simulink model "threeDOFmodel"  (R2018b)
settings: Solver=VariableStepAuto  StartTime=0.0  StopTime=inf  RelTol=1e-3
libraries: robotlib x15, autolibshared x2
settings Model: Creator=ckreienk  LastModifiedBy=ckreienk

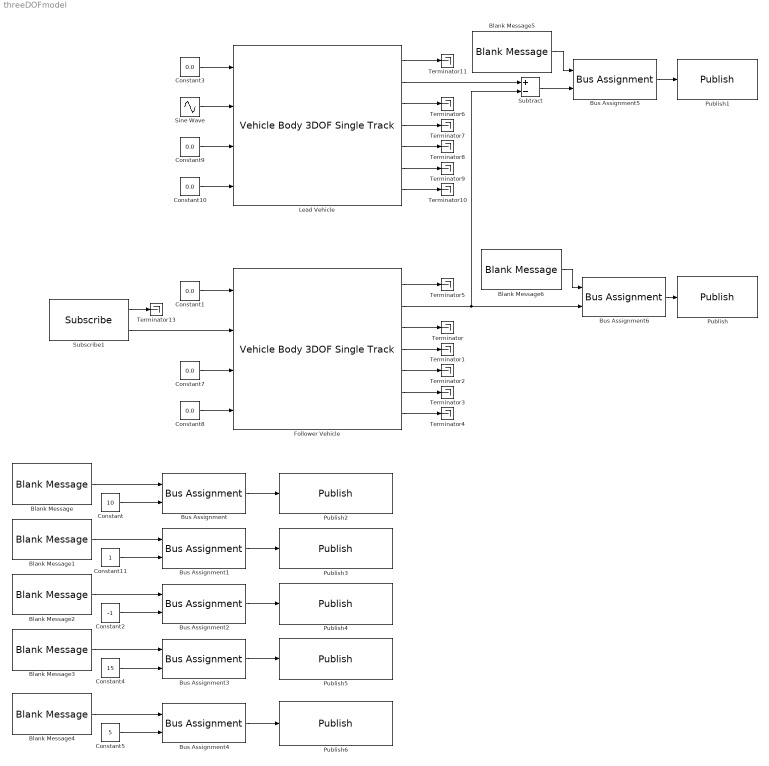
== system threeDOFmodel ==
  Blank Message{,1..6} (7 alike) : robotlib/Blank Message  messageClass=Message  entityType=geometry_msgs/Point  messageType=geometry_msgs/Point  SampleTime=inf
      settings: SourceProductBaseCode=RO
  Bus Assignment{,1..6} (7 alike) : BusAssignment  AssignedSignals=X
  Constant : Constant  Value=10
  Constant{1,3,7..10} (6 alike) : Constant  Value=0.0
  Constant11 : Constant
  Constant2 : Constant  Value=-1
  Constant4 : Constant  Value=15
  Constant5 : Constant  Value=5
  Follower Vehicle : autolibshared/Vehicle Body 3DOF Single Track  trackMode=Dual  inputMode=External longitudinal velocity  frontSteerMode=on  rearSteerMode=off  windMode=off  muMode=on  extFMode=on  extMMode=off  aMode=2  NF=2  NR=2  m=2000  a=1.4  b=1.6  h=0.35  X_o=0  xdot_o=0  CalphaMode=off  sigmaMode=on  d=0  w=[1.4,1.4]  Cy_f=12e3  Cy_r=11e3  sigma_f=.1  sigma_r=.1  alpha_f_brk=[-.1 .1]  Cy_f_data=[-9e3 9e3]  alpha_r_brk=[-.1 .1]  Cy_r_data=[-9e3 9e3]  Y_o=0  ydot_o=0  Izz=4000  psi_o=0  r_o=0  Af=2  Cd=.3  Cl=.1  Cpm=.1  beta_w=[0:0.01:0.3]  Cs=[0:0.03:0.9]  Cym=[0:0.01:0.3]  Pabs=101325  Tair=273  g=9.81  mu=1  xdot_tol=.01  Fznom=5000  Fxtire_sat=7e4  Fytire_sat=7e4  longOff=0  latOff=0  vertOff=0
      settings: SourceProductName=Powertrain Blockset  SourceProductBaseCode=PW
  Lead Vehicle : autolibshared/Vehicle Body 3DOF Single Track  trackMode=Dual  inputMode=External longitudinal velocity  frontSteerMode=on  rearSteerMode=off  windMode=off  muMode=on  extFMode=on  extMMode=off  aMode=2  NF=2  NR=2  m=2000  a=1.4  b=1.6  h=0.35  X_o=0  xdot_o=0  CalphaMode=off  sigmaMode=on  d=0  w=[1.4,1.4]  Cy_f=12e3  Cy_r=11e3  sigma_f=.1  sigma_r=.1  alpha_f_brk=[-.1 .1]  Cy_f_data=[-9e3 9e3]  alpha_r_brk=[-.1 .1]  Cy_r_data=[-9e3 9e3]  Y_o=0  ydot_o=0  Izz=4000  psi_o=0  r_o=0  Af=2  Cd=.3  Cl=.1  Cpm=.1  beta_w=[0:0.01:0.3]  Cs=[0:0.03:0.9]  Cym=[0:0.01:0.3]  Pabs=101325  Tair=273  g=9.81  mu=1  xdot_tol=.01  Fznom=5000  Fxtire_sat=7e4  Fytire_sat=7e4  longOff=0  latOff=0  vertOff=0
      settings: SourceProductName=Powertrain Blockset  SourceProductBaseCode=PW
  Publish : robotlib/Publish  topicSource=Specify your own  topic=vel  messageType=geometry_msgs/Point  messageQueueLength=1
      settings: SourceProductBaseCode=RO
  Publish1 : robotlib/Publish  topicSource=Specify your own  topic=kalmanFilter/vel  messageType=geometry_msgs/Point  messageQueueLength=1
      settings: SourceProductBaseCode=RO
  Publish2 : robotlib/Publish  topicSource=Specify your own  topic=/smoothupparams/max_speed  messageType=geometry_msgs/Point  messageQueueLength=1
      settings: SourceProductBaseCode=RO
  Publish3 : robotlib/Publish  topicSource=Specify your own  topic=/smoothupparams/max_accel  messageType=geometry_msgs/Point  messageQueueLength=1
      settings: SourceProductBaseCode=RO
  Publish4 : robotlib/Publish  topicSource=Specify your own  topic=/smoothupparams/max_decel  messageType=geometry_msgs/Point  messageQueueLength=1
      settings: SourceProductBaseCode=RO
  Publish5 : robotlib/Publish  topicSource=Specify your own  topic=reference_vel  messageType=geometry_msgs/Point  messageQueueLength=1
      settings: SourceProductBaseCode=RO
  Publish6 : robotlib/Publish  topicSource=Specify your own  topic=kalmanFilter/dist  messageType=geometry_msgs/Point  messageQueueLength=1
      settings: SourceProductBaseCode=RO
  Sine Wave : Sin  Amplitude=3  Bias=3  Frequency=3  SampleTime=0
  Subscribe1 : robotlib/Subscribe  topicSource=Specify your own  topic=cmd_vel_wrench  messageType=geometry_msgs/Point  sampleTime=-1  messageQueueLength=1
      settings: SourceProductBaseCode=RO
  Subtract : Sum  Inputs=+-
  Terminator{,1..11,13} (13 alike) : Terminator
  wires:
  Subscribe1/2 -> Follower Vehicle/2
  Constant1/1 -> Follower Vehicle/1
  Follower Vehicle/7 -> Terminator4/1
  Follower Vehicle/6 -> Terminator3/1
  Follower Vehicle/5 -> Terminator2/1
  Follower Vehicle/4 -> Terminator1/1
  Follower Vehicle/3 -> Terminator/1
  Follower Vehicle/1 -> Terminator5/1
  Lead Vehicle/1 -> Terminator11/1
  Lead Vehicle/3 -> Terminator6/1
  Lead Vehicle/4 -> Terminator7/1
  Lead Vehicle/5 -> Terminator8/1
  Lead Vehicle/6 -> Terminator9/1
  Lead Vehicle/7 -> Terminator10/1
  Constant3/1 -> Lead Vehicle/1
  Subscribe1/1 -> Terminator13/1
  Sine Wave/1 -> Lead Vehicle/2
  Bus Assignment5/1 -> Publish1/1
  Constant7/1 -> Follower Vehicle/3
  Constant8/1 -> Follower Vehicle/4
  Constant9/1 -> Lead Vehicle/3
  Constant10/1 -> Lead Vehicle/4
  Bus Assignment/1 -> Publish2/1
  Blank Message/1 -> Bus Assignment/1
  Constant/1 -> Bus Assignment/2
  Constant11/1 -> Bus Assignment1/2
  Blank Message1/1 -> Bus Assignment1/1
  Constant2/1 -> Bus Assignment2/2
  Constant4/1 -> Bus Assignment3/2
  Constant5/1 -> Bus Assignment4/2
  Bus Assignment4/1 -> Publish6/1
  Blank Message4/1 -> Bus Assignment4/1
  Blank Message3/1 -> Bus Assignment3/1
  Blank Message2/1 -> Bus Assignment2/1
  Bus Assignment2/1 -> Publish4/1
  Bus Assignment3/1 -> Publish5/1
  Bus Assignment1/1 -> Publish3/1
  Blank Message5/1 -> Bus Assignment5/1
  Lead Vehicle/2 -> Subtract/1
  Subtract/1 -> Bus Assignment5/2
  Follower Vehicle/2 -> Bus Assignment6/2, Subtract/2
  Blank Message6/1 -> Bus Assignment6/1
  Bus Assignment6/1 -> Publish/1
